simulink model "DrishtiCare_DistrictScreening"  (R2026a)
settings: Solver=FixedStepDiscrete  StopTime=249  FixedStep=1
PreLoadFcn:
  | drishti_sim_default_params
InitFcn:
  | drishti_sim_default_params
undefined symbols (not defined in the file or in its folder): sim_patientsPerDay, sim_prevalence, sim_qFail, sim_qUsable, sim_recapture, sim_sens, sim_spec, sim_specCapacity
settings Model: Creator=aryan  LastModifiedBy=aryan

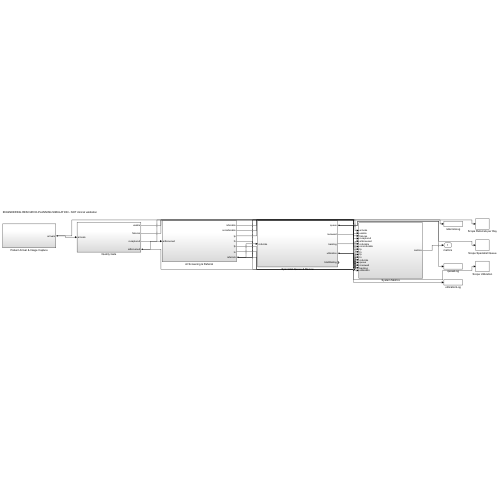
[thumbnail: Simulink's stored preview of the top-level diagram]
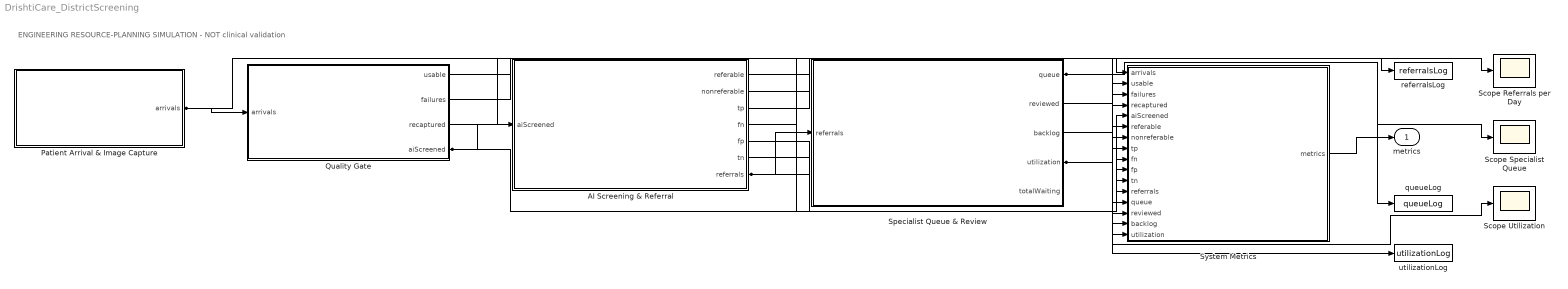
== system DrishtiCare_DistrictScreening ==
  note: ENGINEERING RESOURCE-PLANNING SIMULATION - NOT clinical validation
  AI Screening & Referral : Subsystem
  Patient Arrival & Image Capture : Subsystem
  Quality Gate : Subsystem
  Scope Referrals per Day : Scope
  Scope Specialist Queue : Scope
  Scope Utilization : Scope
  Specialist Queue & Review : Subsystem
  System Metrics : Subsystem
  queueLog : ToWorkspace  VariableName=queueLog
  referralsLog : ToWorkspace  VariableName=referralsLog
  utilizationLog : ToWorkspace  VariableName=utilizationLog
  metrics : Outport
  wires:
  Patient Arrival & Image Capture/1(arrivals) -> Quality Gate/1(arrivals), System Metrics/1(arrivals)
  Quality Gate/4(aiScreened) -> AI Screening & Referral/1(aiScreened), System Metrics/5(aiScreened)
  AI Screening & Referral/7(referrals) -> Specialist Queue & Review/1(referrals), System Metrics/12(referrals), referralsLog/1, Scope Referrals per Day/1
  Quality Gate/1(usable) -> System Metrics/2(usable)
  Quality Gate/2(failures) -> System Metrics/3(failures)
  Quality Gate/3(recaptured) -> System Metrics/4(recaptured)
  AI Screening & Referral/1(referable) -> System Metrics/6(referable)
  AI Screening & Referral/2(nonreferable) -> System Metrics/7(nonreferable)
  AI Screening & Referral/3(tp) -> System Metrics/8(tp)
  AI Screening & Referral/4(fn) -> System Metrics/9(fn)
  AI Screening & Referral/5(fp) -> System Metrics/10(fp)
  AI Screening & Referral/6(tn) -> System Metrics/11(tn)
  Specialist Queue & Review/1(queue) -> System Metrics/13(queue), queueLog/1, Scope Specialist Queue/1
  Specialist Queue & Review/2(reviewed) -> System Metrics/14(reviewed)
  Specialist Queue & Review/3(backlog) -> System Metrics/15(backlog)
  Specialist Queue & Review/4(utilization) -> System Metrics/16(utilization), utilizationLog/1, Scope Utilization/1
  System Metrics/1(metrics) -> metrics/1

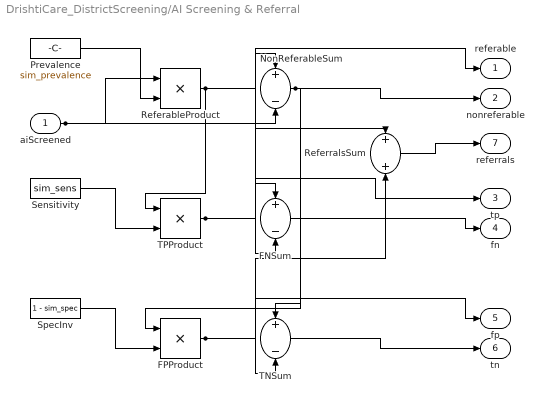
== system DrishtiCare_DistrictScreening/AI Screening & Referral ==
  aiScreened : Inport
  FNSum : Sum  Inputs=+-
  FPProduct : Product
  NonReferableSum : Sum  Inputs=+-
  Prevalence : Constant  Value=sim_prevalence
  ReferableProduct : Product
  ReferralsSum : Sum
  Sensitivity : Constant  Value=sim_sens
  SpecInv : Constant  Value=1 - sim_spec
  TNSum : Sum  Inputs=+-
  TPProduct : Product
  referable : Outport
  nonreferable : Outport  Port=2
  tp : Outport  Port=3
  fn : Outport  Port=4
  fp : Outport  Port=5
  tn : Outport  Port=6
  referrals : Outport  Port=7
  wires:
  aiScreened/1 -> ReferableProduct/1, NonReferableSum/1
  Prevalence/1 -> ReferableProduct/2
  ReferableProduct/1 -> NonReferableSum/2, TPProduct/1, FNSum/1, referable/1
  Sensitivity/1 -> TPProduct/2
  TPProduct/1 -> FNSum/2, ReferralsSum/1, tp/1
  NonReferableSum/1 -> FPProduct/1, TNSum/1, nonreferable/1
  SpecInv/1 -> FPProduct/2
  FPProduct/1 -> TNSum/2, ReferralsSum/2, fp/1
  FNSum/1 -> fn/1
  TNSum/1 -> tn/1
  ReferralsSum/1 -> referrals/1

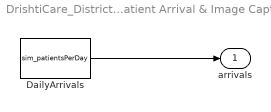
== system DrishtiCare_DistrictScreening/Patient Arrival & Image Capture ==
  DailyArrivals : Constant  Value=sim_patientsPerDay
  arrivals : Outport
  wires:
  DailyArrivals/1 -> arrivals/1

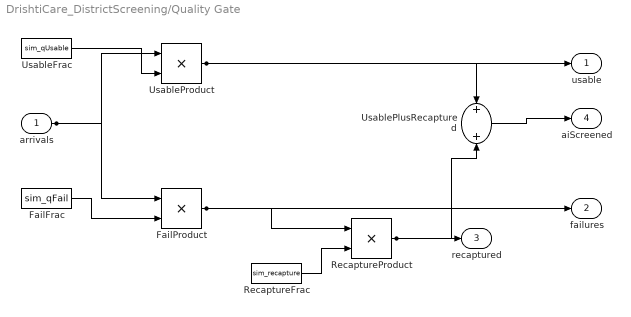
== system DrishtiCare_DistrictScreening/Quality Gate ==
  arrivals : Inport
  FailFrac : Constant  Value=sim_qFail
  FailProduct : Product
  RecaptureFrac : Constant  Value=sim_recapture
  RecaptureProduct : Product
  UsableFrac : Constant  Value=sim_qUsable
  UsablePlusRecaptured : Sum
  UsableProduct : Product
  usable : Outport
  failures : Outport  Port=2
  recaptured : Outport  Port=3
  aiScreened : Outport  Port=4
  wires:
  arrivals/1 -> UsableProduct/1, FailProduct/1
  UsableFrac/1 -> UsableProduct/2
  FailFrac/1 -> FailProduct/2
  FailProduct/1 -> RecaptureProduct/1, failures/1
  RecaptureFrac/1 -> RecaptureProduct/2
  UsableProduct/1 -> UsablePlusRecaptured/1, usable/1
  RecaptureProduct/1 -> UsablePlusRecaptured/2, recaptured/1
  UsablePlusRecaptured/1 -> aiScreened/1

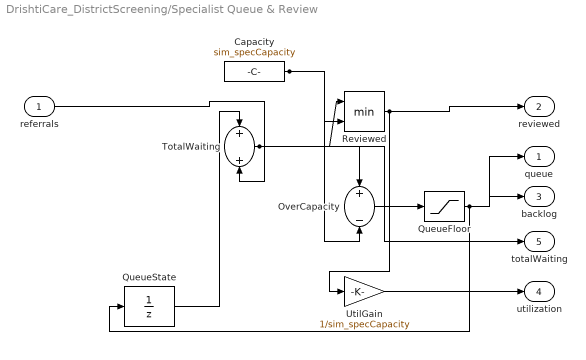
== system DrishtiCare_DistrictScreening/Specialist Queue & Review ==
  referrals : Inport
  Capacity : Constant  Value=sim_specCapacity
  OverCapacity : Sum  Inputs=+-
  QueueFloor : Saturate  UpperLimit=inf  LowerLimit=0
  QueueState : UnitDelay
  Reviewed : MinMax  Inputs=2
  TotalWaiting : Sum
  UtilGain : Gain  Gain=1/sim_specCapacity
  queue : Outport
  reviewed : Outport  Port=2
  backlog : Outport  Port=3
  utilization : Outport  Port=4
  totalWaiting : Outport  Port=5
  wires:
  QueueState/1 -> TotalWaiting/1
  referrals/1 -> TotalWaiting/2
  TotalWaiting/1 -> Reviewed/1, OverCapacity/1, totalWaiting/1
  Capacity/1 -> Reviewed/2, OverCapacity/2
  OverCapacity/1 -> QueueFloor/1
  QueueFloor/1 -> QueueState/1, queue/1, backlog/1
  Reviewed/1 -> UtilGain/1, reviewed/1
  UtilGain/1 -> utilization/1

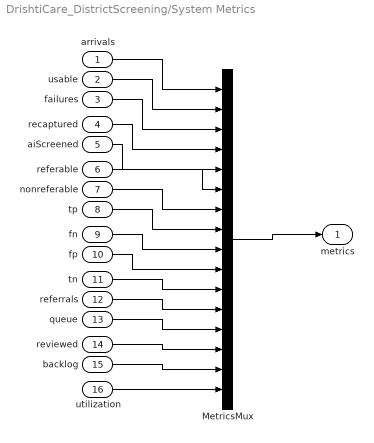
== system DrishtiCare_DistrictScreening/System Metrics ==
  arrivals : Inport
  usable : Inport  Port=2
  failures : Inport  Port=3
  recaptured : Inport  Port=4
  aiScreened : Inport  Port=5
  referable : Inport  Port=6
  nonreferable : Inport  Port=7
  tp : Inport  Port=8
  fn : Inport  Port=9
  fp : Inport  Port=10
  tn : Inport  Port=11
  referrals : Inport  Port=12
  queue : Inport  Port=13
  reviewed : Inport  Port=14
  backlog : Inport  Port=15
  utilization : Inport  Port=16
  MetricsMux : Mux  Inputs=16
  metrics : Outport
  wires:
  arrivals/1 -> MetricsMux/1
  usable/1 -> MetricsMux/2
  failures/1 -> MetricsMux/3
  recaptured/1 -> MetricsMux/4
  aiScreened/1 -> MetricsMux/5
  referable/1 -> MetricsMux/6
  nonreferable/1 -> MetricsMux/7
  tp/1 -> MetricsMux/8
  fn/1 -> MetricsMux/9
  fp/1 -> MetricsMux/10
  tn/1 -> MetricsMux/11
  referrals/1 -> MetricsMux/12
  queue/1 -> MetricsMux/13
  reviewed/1 -> MetricsMux/14
  backlog/1 -> MetricsMux/15
  utilization/1 -> MetricsMux/16
  MetricsMux/1 -> metrics/1
